simulink model "Tirocinio3Simulink2"  (R2025b)
settings: Solver=VariableStepAuto  StartTime=0.0  StopTime=10.0  RelTol=1e-3
undefined symbols (not defined in the file or in its folder): A_cplx, A_real_cplx, B_cplx, B_real_cplx, C_cplx, C_real_cplx, H_fast_cplx, H_kalman_cplx, H_slow_cplx, M_cplx, R_cplx, V_fast_cplx, V_kalman_cplx, V_slow_cplx
libraries: simulink x1
settings Model: Creator=Davide  LastModifiedBy=Davide

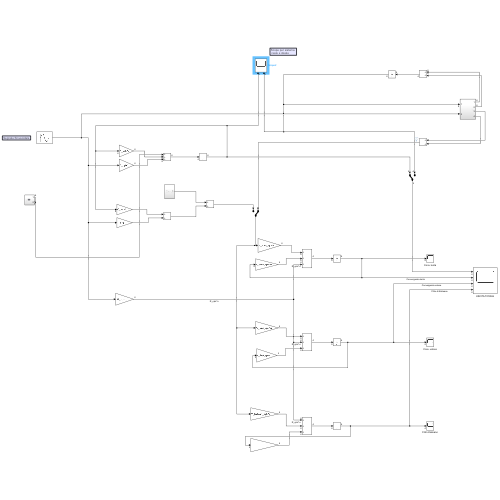
[thumbnail: Simulink's stored preview of the top-level diagram]
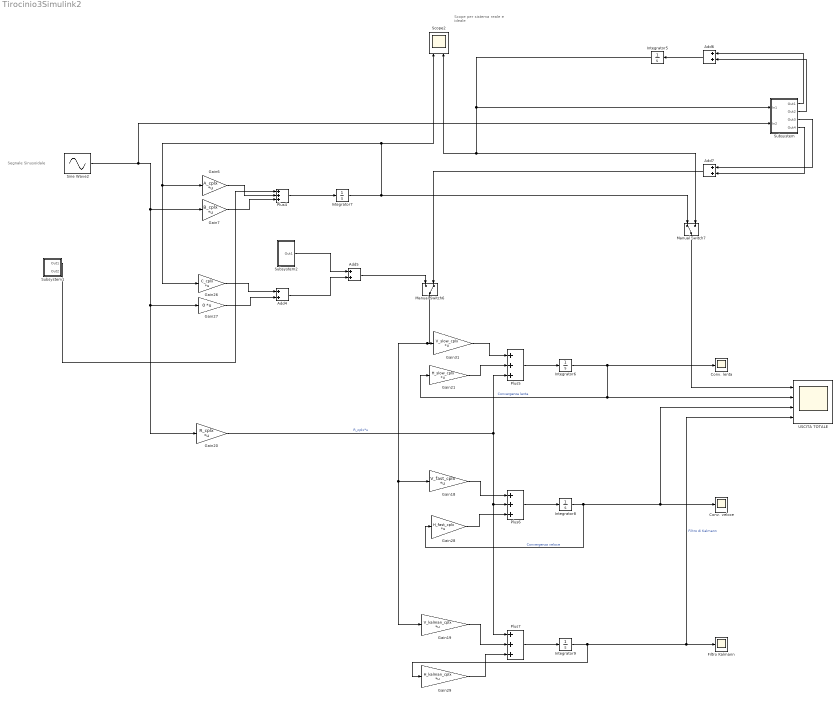
== system Tirocinio3Simulink2 ==
  note: Segnale Sinusoidale
  note: Scope per sistema
      |  reale e ideale
  Add{4..7} (4 alike) : Sum
  Conv. lenta : Scope
      settings: ActiveDisplayYMinimum=-8.74771  ActiveDisplayYMaximum=8.48508
  Conv. veloce : Scope
      settings: ActiveDisplayYMinimum=-1.73756  ActiveDisplayYMaximum=6.44374  DataLoggingVariableName=ScopeData2
  "Filtro Kalmann " : Scope
      settings: ActiveDisplayYMinimum=-0.72619  ActiveDisplayYMaximum=4.40922  DataLoggingVariableName=ScopeData3
  Gain18 : Gain  Gain=V_fast_cplx  Multiplication=Matrix(K*u)
  Gain19 : Gain  Gain=V_kalman_cplx  Multiplication=Matrix(K*u)
  Gain20 : Gain  Gain=R_cplx  Multiplication=Matrix(K*u)
  Gain21 : Gain  Gain=H_slow_cplx  Multiplication=Matrix(K*u)
  Gain26 : Gain  Gain=C_cplx  Multiplication=Matrix(K*u)
  Gain27 : Gain  Gain=0  Multiplication=Matrix(K*u)
  Gain28 : Gain  Gain=H_fast_cplx  Multiplication=Matrix(K*u)
  Gain29 : Gain  Gain=H_kalman_cplx  Multiplication=Matrix(K*u)
  Gain31 : Gain  Gain=V_slow_cplx  Multiplication=Matrix(K*u)
  Gain6 : Gain  Gain=A_cplx  Multiplication=Matrix(K*u)
  Gain7 : Gain  Gain=B_cplx  Multiplication=Matrix(K*u)
  Integrator5 : Integrator  AbsoluteTolerance=1
  Integrator6 : Integrator  InitialCondition=0.2  AbsoluteTolerance=1
  Integrator7 : Integrator  InitialCondition=0.1  AbsoluteTolerance=1
  Integrator8 : Integrator  InitialCondition=0.2  AbsoluteTolerance=1
  Integrator9 : Integrator  InitialCondition=0.2  AbsoluteTolerance=1
  Manual Switch6 : ManualSwitch  CurrentSetting=0
  Manual Switch7 : ManualSwitch
  Plus{4..7} (4 alike) : Sum  Inputs=+++
  Scope2 : Scope  NumInputPorts=2
      settings: Title=Parametri Reali  ActiveDisplayYMinimum=-3.1392104169131572  ActiveDisplayYMaximum=6.0573480578115992  DataLoggingVariableName=ScopeData4
  Sine Wave2 : Sin  SampleTime=0
  Subsystem : Subsystem
  Subsystem1 : Subsystem
  Subsystem2 : Subsystem
  USCITA TOTALE : Scope  NumInputPorts=4
      settings: ActiveDisplayString=3  ActiveDisplayYMinimum=-0.5390835365986395  ActiveDisplayYMaximum=4.4422634634013622  DataLoggingVariableName=ScopeData5
  wires:
  Manual Switch7/1 -> USCITA TOTALE/1
  Gain7/1 -> Plus4/3
  Plus4/1 -> Integrator7/1
  Gain21/1 -> Plus5/2
  Gain28/1 -> Plus6/3
  Gain20/1 -> Plus5/3, Plus7/1, Plus6/2  "R_cplx*u"
  Gain29/1 -> Plus7/3
  Integrator6/1 -> Gain21/1, USCITA TOTALE/2, Conv. lenta/1  "Convergenza lenta"
  Integrator9/1 -> Gain29/1, "Filtro Kalmann "/1, USCITA TOTALE/4  "Filtro di Kalmann"
  Gain19/1 -> Plus7/2
  Gain18/1 -> Plus6/1
  Add7/1 -> Manual Switch6/2
  Integrator7/1 -> Gain26/1, Gain6/1, Scope2/1, Manual Switch7/1
  Gain31/1 -> Plus5/1
  Add4/1 -> Add5/2
  Plus6/1 -> Integrator8/1
  Gain27/1 -> Add4/2
  Integrator5/1 -> Scope2/2, Manual Switch7/2, Subsystem/1(In1)
  Manual Switch6/1 -> Gain19/1, Gain18/1, Gain31/1
  Gain6/1 -> Plus4/2
  Gain26/1 -> Add4/1
  Add5/1 -> Manual Switch6/1
  Sine Wave2/1 -> Subsystem/2(In2), Gain20/1, Gain27/1, Gain7/1
  Plus7/1 -> Integrator9/1
  Plus5/1 -> Integrator6/1
  Integrator8/1 -> USCITA TOTALE/3, Conv. veloce/1, Gain28/1  "Convergenza veloce"
  Add6/1 -> Integrator5/1
  Subsystem/1(Out1) -> Add6/1
  Subsystem/2(Out2) -> Add6/2
  Subsystem/3(Out3) -> Add7/1
  Subsystem/4(Out4) -> Add7/2
  Subsystem1/1(Out1) -> Plus4/1
  Subsystem2/1(Out1) -> Add5/1

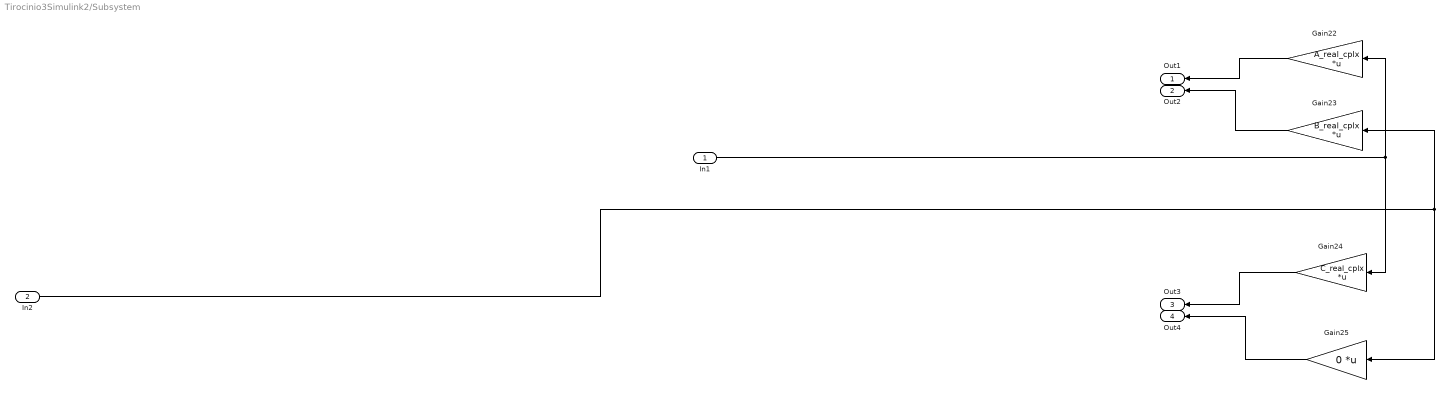
== system Tirocinio3Simulink2/Subsystem ==
  In1 : Inport
  In2 : Inport  Port=2
  Gain22 : Gain  Gain=A_real_cplx  Multiplication=Matrix(K*u)
  Gain23 : Gain  Gain=B_real_cplx  Multiplication=Matrix(K*u)
  Gain24 : Gain  Gain=C_real_cplx  Multiplication=Matrix(K*u)
  Gain25 : Gain  Gain=0  Multiplication=Matrix(K*u)
  Out1 : Outport
  Out2 : Outport  Port=2
  Out3 : Outport  Port=3
  Out4 : Outport  Port=4
  wires:
  Gain25/1 -> Out4/1
  In2/1 -> Gain25/1, Gain23/1
  Gain22/1 -> Out1/1
  Gain24/1 -> Out3/1
  In1/1 -> Gain24/1, Gain22/1
  Gain23/1 -> Out2/1

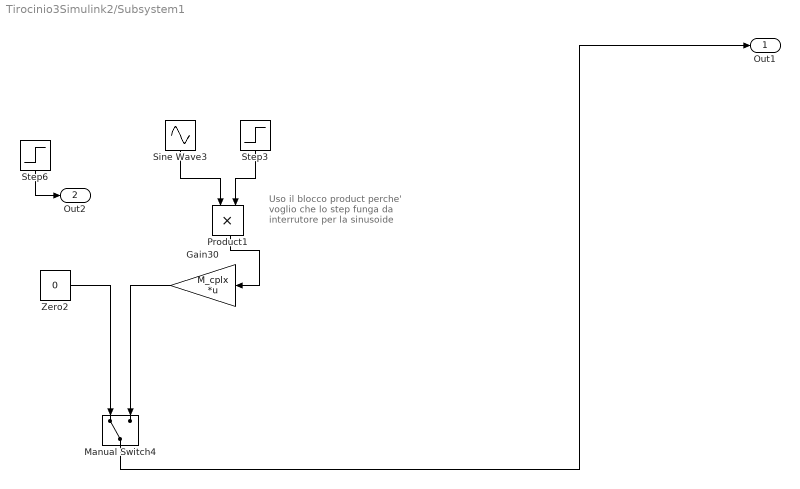
== system Tirocinio3Simulink2/Subsystem1 ==
  note: Uso il blocco product
      | perche' voglio che lo step
      | funga da interrutore per la
      | sinusoide
  Gain30 : Gain  Gain=M_cplx  Multiplication=Matrix(K*u)
  Manual Switch4 : ManualSwitch
  Product1 : Product
  Sine Wave3 : Sin  SampleTime=0
  Step3 : Step  SampleTime=0
  Step6 : Step  SampleTime=0
  Zero2 : Constant  Value=0  OutDataTypeStr=Inherit: Inherit via back propagation
  Out1 : Outport
  Out2 : Outport  Port=2
  wires:
  Product1/1 -> Gain30/1
  Manual Switch4/1 -> Out1/1
  Gain30/1 -> Manual Switch4/2
  Sine Wave3/1 -> Product1/1
  Step6/1 -> Out2/1
  Zero2/1 -> Manual Switch4/1
  Step3/1 -> Product1/2

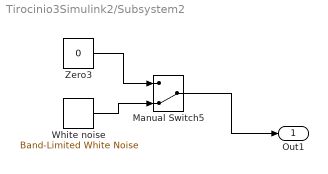
== system Tirocinio3Simulink2/Subsystem2 ==
  Manual Switch5 : ManualSwitch  CurrentSetting=0
  White noise : simulink/Sources/Band-Limited White Noise  Cov=[0.1]  Ts=0.1  seed=[23341]
  Zero3 : Constant  Value=0  OutDataTypeStr=Inherit: Inherit via back propagation
  Out1 : Outport
  wires:
  Zero3/1 -> Manual Switch5/1
  White noise/1 -> Manual Switch5/2
  Manual Switch5/1 -> Out1/1
